simulink model "simulation_discrete"  (R2024b)
settings: Solver=FixedStepAuto  StartTime=0.0  StopTime=30  FixedStep=Ts  RelTol=1e-3
values from neighbouring files (symbols this model uses):
  output_position_power = 0.005    [main_discrete.m]
  P0 = 2*Q    [main_discrete.m]
  real_inital_position = [-0.4;0.3]    [main_discrete.m]
  real_inital_r = -0.2    [main_discrete.m]
  real_inital_surge = 5    [main_discrete.m]
  real_inital_yaw = pi/2    (= 1.57079632679)    [main_discrete.m]
  sim_data = struct    [main_discrete.m]
  state0_hat = [initial_x_estimate; initial_y_estimate; initial_surge_estimate; initial_yaw_estimate; initial_r_estimate]    [main_discrete.m]
  use_position_noise = 1    [main_discrete.m]
libraries: simulink x2
settings Model: Creator=ricar  LastModifiedBy=ricar

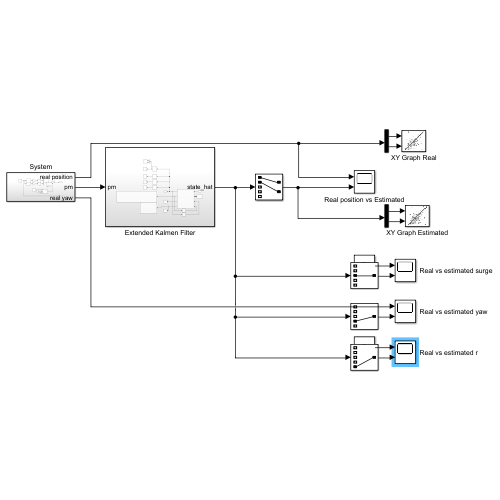
[thumbnail: Simulink's stored preview of the top-level diagram]
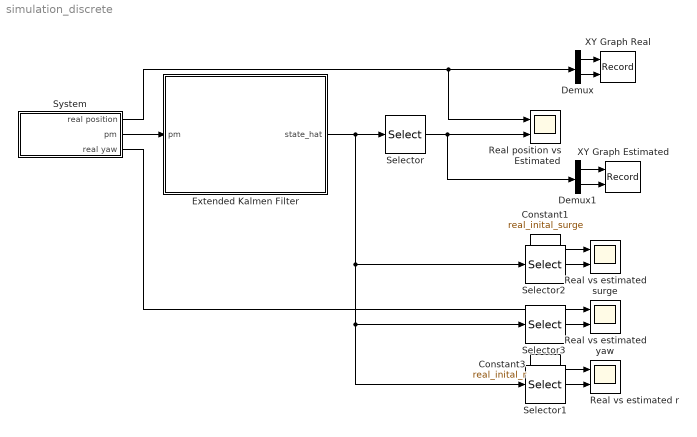
== system simulation_discrete ==
  Constant1 : Constant  Value=real_inital_surge
  Constant3 : Constant  Value=real_inital_r
  Demux : Demux  Outputs=2
  Demux1 : Demux  Outputs=2
  Extended Kalmen Filter : Subsystem
  Real position vs Estimated : Scope  NumInputPorts=2
  Real vs estimated r : Scope  NumInputPorts=2
  Real vs estimated surge : Scope  NumInputPorts=2
  Real vs estimated yaw : Scope  NumInputPorts=2
  Selector : Selector  InputPortWidth=5  IndexOptions=Index vector (dialog)  Indices=[1 2]  OutputSizes=1
  Selector1 : Selector  InputPortWidth=5  IndexOptions=Index vector (dialog)  Indices=[5]  OutputSizes=1
  Selector2 : Selector  InputPortWidth=5  IndexOptions=Index vector (dialog)  Indices=[3]  OutputSizes=1
  Selector3 : Selector  InputPortWidth=5  IndexOptions=Index vector (dialog)  Indices=[4]  OutputSizes=1
  System : Subsystem
  XY Graph Estimated : Record  FileSettingsInternal="{\"entries\":[{\"content\":{\"excelSettings\":{\"content\":{},\"type\":\"Streamout.ExcelSettings\"}},\"type\":\"Streamout.FileSettingStorage\",\"uuid\":\"\"}],\"packageUris\":[\"http:\\/\\/schema.mathworks.com\\/mf0\\/streamout_blocks\\/R2020a\"],\"version\":\"1.0\"}"  Layout=[1 1]  SignalsInternal="{\"entries\":[{\"content\":{\"signals\":[{\"content\":{\"blockPath\":[],\"dimensions\":[1,1],\"domain\":\"\",\"lineColor\":\"#a2142f\",\"plots\":[ 1 ],\"port\":1,\"sid\":[\"\"],\"signalID\":1,\"signalName\":\"Demux1:1\"},\"type\":\"RecordBlkView.Signal\",\"uuid\":\"\"},{\"content\":{\"blockPath\":[],\"dimensions\":[1,1],\"domain\":\"\",\"lineColor\":\"#139fff\",\"plots\":[ 1 ],\"port\":2,\"sid\":[\"\"],\"signalID\":2,\"signalName\":\"Demux1:2\"},\"type\":\"RecordBlkView.Signal\",\"uuid\":\"\"}]},\"type\":\"RecordBlkView.InputSignals\",\"uuid\":\"\"}],\"packageUris\":[\"http:\\/\\/schema.mathworks.com\\/mf0\\/streamout_blocks\\/R2020a\"],\"version\":\"1.0\"}"  VisualizationBindings="{\"xyplotplugin\":{\"info\":[{\"series\":[{\"bindingParametersList\":[{\"parameter\":\"X-Axis\",\"signalID\":1,\"signalName\":\"Demux1:1\"},{\"parameter\":\"Y-Axis\",\"signalID\":2,\"signalName\":\"Demux1:2\"}],\"seriesID\":0}],\"subplotID\":1}]}}"  CompatibilityTag=XY
  XY Graph Real : Record  FileSettingsInternal="{\"entries\":[{\"content\":{\"excelSettings\":{\"content\":{},\"type\":\"Streamout.ExcelSettings\"}},\"type\":\"Streamout.FileSettingStorage\",\"uuid\":\"\"}],\"packageUris\":[\"http:\\/\\/schema.mathworks.com\\/mf0\\/streamout_blocks\\/R2020a\"],\"version\":\"1.0\"}"  Layout=[1 1]  SignalsInternal="{\"entries\":[{\"content\":{\"signals\":[{\"content\":{\"blockPath\":[],\"dimensions\":[1],\"domain\":\"\",\"lineColor\":\"#64d413\",\"lineWidth\":2,\"plots\":[ 1 ],\"port\":1,\"sid\":[\"\"],\"signalID\":1,\"signalName\":\"Demux:1\"},\"type\":\"RecordBlkView.Signal\",\"uuid\":\"\"},{\"content\":{\"blockPath\":[],\"dimensions\":[1],\"domain\":\"\",\"lineColor\":\"#ff13a6\",\"lineWidth\":2,\"plots\":[ 1 ],\"port\":2,\"sid\":[\"\"],\"signalID\":2,\"signalName\":\"Demux:2\"},\"type\":\"RecordBlkView.Signal\",\"uuid\":\"\"}]},\"type\":\"RecordBlkView.InputSignals\",\"uuid\":\"\"}],\"packageUris\":[\"http:\\/\\/schema.mathworks.com\\/mf0\\/streamout_blocks\\/R2020a\"],\"version\":\"1.0\"}"  VisualizationBindings="{\"xyplotplugin\":{\"info\":[{\"series\":[{\"bindingParametersList\":[{\"parameter\":\"X-Axis\",\"signalID\":1,\"signalName\":\"Demux:1\"},{\"parameter\":\"Y-Axis\",\"signalID\":2,\"signalName\":\"Demux:2\"}],\"seriesID\":0}],\"subplotID\":1}]}}"  CompatibilityTag=XY
  wires:
  System/2(pm) -> Extended Kalmen Filter/1(pm)
  Extended Kalmen Filter/1(state_hat) -> Selector3/1, Selector1/1, Selector2/1, Selector/1
  System/1(real position) -> Real position vs Estimated/1, Demux/1
  Selector/1 -> Demux1/1, Real position vs Estimated/2
  Demux1/2 -> XY Graph Estimated/2
  Demux1/1 -> XY Graph Estimated/1
  Demux/1 -> XY Graph Real/1
  Demux/2 -> XY Graph Real/2
  Constant1/1 -> Real vs estimated surge/1
  Selector2/1 -> Real vs estimated surge/2
  Selector3/1 -> Real vs estimated yaw/2
  System/3(real yaw) -> Real vs estimated yaw/1
  Selector1/1 -> Real vs estimated r/2
  Constant3/1 -> Real vs estimated r/1

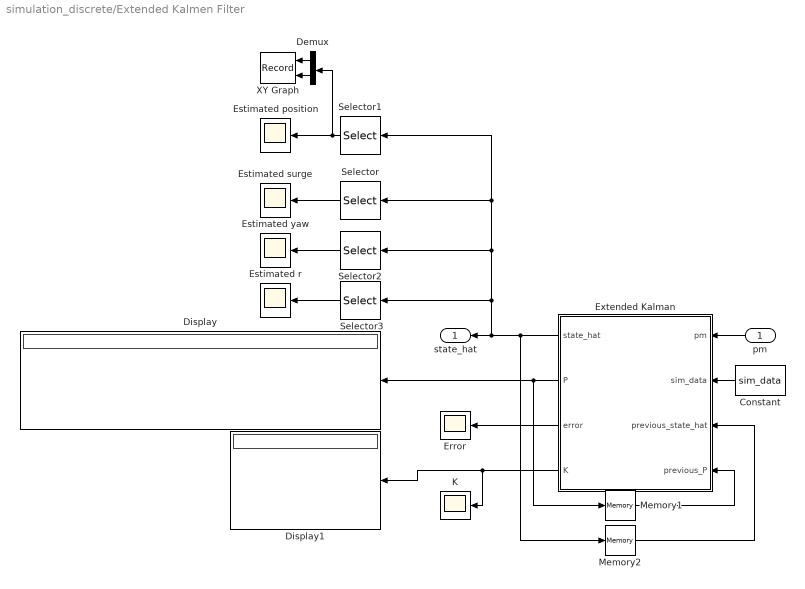
== system simulation_discrete/Extended Kalmen Filter ==
  pm : Inport
  Constant : Constant  Value=sim_data  OutDataTypeStr=Bus: busObject
  Demux : Demux  Outputs=2
  Display : Display
  Display1 : Display
  Error : Scope
  Estimated position : Scope
  Estimated r : Scope
  Estimated surge : Scope
  Estimated yaw : Scope
  Extended Kalman : MATLAB Function  TreatAsAtomicUnit=on
  K : Scope
  Memory1 : Memory  InitialCondition=P0
  Memory2 : Memory  InitialCondition=state0_hat
  Selector : Selector  InputPortWidth=5  IndexOptions=Index vector (dialog)  Indices=[3]  OutputSizes=1
  Selector1 : Selector  InputPortWidth=5  IndexOptions=Index vector (dialog)  Indices=[1 2]  OutputSizes=1
  Selector2 : Selector  InputPortWidth=5  IndexOptions=Index vector (dialog)  Indices=[4]  OutputSizes=1
  Selector3 : Selector  InputPortWidth=5  IndexOptions=Index vector (dialog)  Indices=[5]  OutputSizes=1
  XY Graph : Record  FileSettingsInternal="{\"entries\":[{\"content\":{\"excelSettings\":{\"content\":{},\"type\":\"Streamout.ExcelSettings\"}},\"type\":\"Streamout.FileSettingStorage\",\"uuid\":\"\"}],\"packageUris\":[\"http:\\/\\/schema.mathworks.com\\/mf0\\/streamout_blocks\\/R2020a\"],\"version\":\"1.0\"}"  Layout=[1 1]  SignalsInternal="{\"entries\":[{\"content\":{\"signals\":[{\"content\":{\"blockPath\":[],\"dimensions\":[1,1],\"domain\":\"\",\"lineColor\":\"#fe330a\",\"lineWidth\":2,\"plots\":[ 1 ],\"port\":1,\"sid\":[\"\"],\"signalID\":1,\"signalName\":\"Demux:1\"},\"type\":\"RecordBlkView.Signal\",\"uuid\":\"\"},{\"content\":{\"blockPath\":[],\"dimensions\":[1,1],\"domain\":\"\",\"lineColor\":\"#22b573\",\"lineWidth\":2,\"plots\":[ 1 ],\"port\":2,\"sid\":[\"\"],\"signalID\":2,\"signalName\":\"Demux:2\"},\"type\":\"RecordBlkView.Signal\",\"uuid\":\"\"}]},\"type\":\"RecordBlkView.InputSignals\",\"uuid\":\"\"}],\"packageUris\":[\"http:\\/\\/schema.mathworks.com\\/mf0\\/streamout_blocks\\/R2020a\"],\"version\":\"1.0\"}"  VisualizationBindings="{\"xyplotplugin\":{\"info\":[{\"series\":[{\"bindingParametersList\":[{\"parameter\":\"X-Axis\",\"signalID\":1,\"signalName\":\"Demux:1\"},{\"parameter\":\"Y-Axis\",\"signalID\":2,\"signalName\":\"Demux:2\"}],\"seriesID\":0},{\"bindingParametersList\":[{\"parameter\":\"X-Axis\",\"signalID\":2,\"signalName\":\"Demux:2\"}],\"seriesID\":1}],\"subplotID\":1}]}}"  CompatibilityTag=XY
  state_hat : Outport
  wires:
  pm/1 -> Extended Kalman/1(pm)
  Constant/1 -> Extended Kalman/2(sim_data)
  Extended Kalman/1(state_hat) -> Memory2/1, state_hat/1, Selector3/1, Selector2/1, Selector1/1, Selector/1
  Memory1/1 -> Extended Kalman/4(previous_P)
  Extended Kalman/2(P) -> Memory1/1, Display/1
  Memory2/1 -> Extended Kalman/3(previous_state_hat)
  Selector1/1 -> Demux/1, Estimated position/1
  Selector/1 -> Estimated surge/1
  Demux/2 -> XY Graph/2
  Demux/1 -> XY Graph/1
  Extended Kalman/4(K) -> Display1/1, K/1
  Selector2/1 -> Estimated yaw/1
  Selector3/1 -> Estimated r/1
  Extended Kalman/3(error) -> Error/1

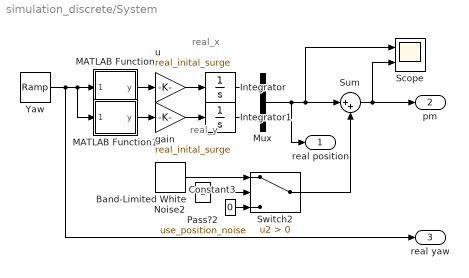
== system simulation_discrete/System ==
  note: real_x
  note: real_y
  Band-Limited White Noise2 : simulink/Sources/Band-Limited White Noise  Cov=[output_position_power,output_position_power]  Ts=0.1  seed=[2,3]
  Constant3 : Constant  Value=0
  Integrator : Integrator  InitialCondition=real_inital_position(1)
  Integrator1 : Integrator  InitialCondition=real_inital_position(2)
  MATLAB Function : MATLAB Function  TreatAsAtomicUnit=on
  MATLAB Function1 : MATLAB Function  TreatAsAtomicUnit=on
  Mux : Mux  Inputs=2
  Pass?2 : Constant  Value=use_position_noise
  Scope : Scope  NumInputPorts=2
  Sum : Sum  Inputs=|++
  Switch2 : Switch  Criteria=u2 > Threshold  SaturateOnIntegerOverflow=off  InputSameDT=off
  Yaw : simulink/Sources/Ramp  slope=real_inital_r  start=0  InitialOutput=real_inital_yaw
  gain : Gain  Gain=real_inital_surge
  u : Gain  Gain=real_inital_surge
  real position : Outport
  pm : Outport  Port=2
  real yaw : Outport  Port=3
  wires:
  Yaw/1 -> MATLAB Function1/1(degrees), MATLAB Function/1(degrees), real yaw/1
  MATLAB Function1/1(y) -> gain/1
  MATLAB Function/1(y) -> u/1
  Constant3/1 -> Switch2/3
  Switch2/1 -> Sum/2
  Band-Limited White Noise2/1 -> Switch2/1
  Pass?2/1 -> Switch2/2
  Mux/1 -> Scope/1, Sum/1, real position/1
  Sum/1 -> Scope/2, pm/1
  u/1 -> Integrator/1
  gain/1 -> Integrator1/1
  Integrator/1 -> Mux/1
  Integrator1/1 -> Mux/2

== matlab function simulation_discrete/System/MATLAB Function ==
  data: degrees input; y output
function y = cosd(degrees)

y = cos(degrees);

== matlab function simulation_discrete/Extended Kalmen Filter/Extended Kalman ==
  data: pm input; sim_data input; state_hat output; previous_state_hat input; previous_P input; P output; error output; K output
function [state_hat, P, error, K] = fcn(pm,sim_data,previous_state_hat,previous_P)

% Initialize variable from workspace
    % Known:

    % System dynamics
    F_linear = sim_data.F;
    H = sim_data.H;
    Ts = sim_data.Ts;

    % Nonlinear dynamics matrix - position calculation
    f_x = @(x,u,yaw) x + u * cos(yaw) * Ts ;
    f_y = @(y,u,yaw) y + u * sin(yaw) * Ts ;
    
    % jacobian of nonlinear output matrix 
    J_f = @(x_hat,y_hat, u_hat, yaw_hat, r_hat) [...
        1, 0, cos(yaw_hat) * Ts, -u_hat * sin(yaw_hat) * Ts, 0; ...
        0, 1, sin(yaw_hat) * Ts, u_hat * cos(yaw_hat) * Ts, 0 ];

    % Filter initiation
    Q = sim_data.state_noise;
    R = sim_data.measurement_noise;
    I = eye(5);

%% Extended Kalmen Filter Logic

x_previous = previous_state_hat(1);
y_previous = previous_state_hat(2);
u_previous = previous_state_hat(3);
yaw_previous = previous_state_hat(4);
r_previous = previous_state_hat(5);

% Linearize dynamics

F_linearized = J_f(x_previous, y_previous, u_previous, yaw_previous, r_previous);

F_full = [F_linearized; F_linear];

% Prediction
prediction_P = F_full * previous_P * F_full'+ Q;

x_prediction = f_x(x_previous,u_previous,yaw_previous);
y_prediction = f_y(y_previous,u_previous,yaw_previous);

state_prediction = F_linear * [x_previous; y_previous; u_previous; yaw_previous; r_previous]; 
state_prediction = [x_prediction; y_prediction; state_prediction];

output_prediction = H * state_prediction;

% Update
K = prediction_P*H'*(H*prediction_P*H' + R)^-1;
error = pm-output_prediction;
state_hat = state_prediction + K*error;

P = (I - (K * H))* prediction_P;

== matlab function simulation_discrete/System/MATLAB Function1 ==
  data: degrees input; y output
function y = sind(degrees)

y = sin(degrees);
